simulink model "dynamiczny_model_ciagly"  (R2021a)
settings: Solver=VariableStepAuto  StartTime=0.0  StopTime=50.0  RelTol=1e-3
settings Model: Creator=48604  LastModifiedBy=48604

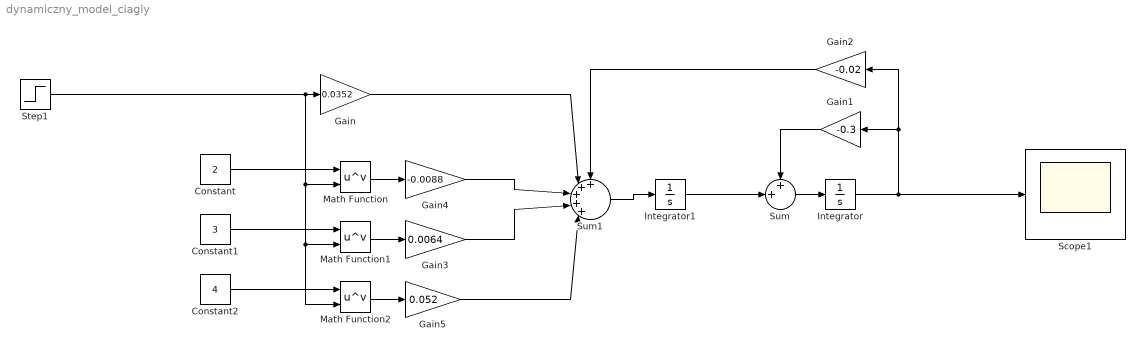
== system dynamiczny_model_ciagly ==
  Constant : Constant  Value=2
  Constant1 : Constant  Value=3
  Constant2 : Constant  Value=4
  Gain : Gain  Gain=0.0352
  Gain1 : Gain  Gain=-0.3
  Gain2 : Gain  Gain=-0.02
  Gain3 : Gain  Gain=0.0064
  Gain4 : Gain  Gain=-0.0088
  Gain5 : Gain  Gain=0.052
  Integrator : Integrator
  Integrator1 : Integrator
  Math Function : Math  Operator=pow  SaturateOnIntegerOverflow=on
  Math Function1 : Math  Operator=pow  SaturateOnIntegerOverflow=on
  Math Function2 : Math  Operator=pow  SaturateOnIntegerOverflow=on
  Scope1 : Scope
  Step1 : Step  SampleTime=0.1
  Sum : Sum  Inputs=++|
  Sum1 : Sum  Inputs=+++++|
  wires:
  Integrator1/1 -> Sum/2
  Sum/1 -> Integrator/1
  Integrator/1 -> Scope1/1, Gain2/1, Gain1/1
  Gain1/1 -> Sum/1
  Sum1/1 -> Integrator1/1
  Math Function1/1 -> Gain3/1
  Math Function2/1 -> Gain5/1
  Constant/1 -> Math Function/1
  Constant1/1 -> Math Function1/1
  Constant2/1 -> Math Function2/1
  Step1/1 -> Math Function2/2, Math Function1/2, Math Function/2, Gain/1
  Gain/1 -> Sum1/2
  Math Function/1 -> Gain4/1
  Gain4/1 -> Sum1/3
  Gain3/1 -> Sum1/4
  Gain5/1 -> Sum1/5
  Gain2/1 -> Sum1/1
